simulink model "sl_lanechange"  (Simulink 7.5)
settings: Solver=ode45  StartTime=0.0  StopTime=10.0  RelTol=1e-3
libraries: simulink x2, roblocks x1
settings Model: Creator=pic  LastModifiedBy=corkep
settings DebuggingCC: StrictBusMsg=Warning

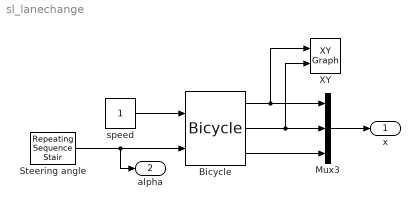
== system sl_lanechange ==
  Bicycle : roblocks/Bicycle  SystemSampleTime=-1  accel=1  vlim=1  alim=2  x0=[0, 0, 0]
  Mux3 : Mux  Inputs=3
  Steering angle : simulink/Sources/Repeating Sequence Stair  SystemSampleTime=-1  OutValues=[0 0 0 0.5 0 -0.5 0 0 0 0]  tsamp=1  OutMin=[]  OutMax=[]  OutDataTypeStr=double  OutputDataTypeScalingMode=Specify via dialog  OutDataType=double  ConRadixGroup=Best Precision: Vector-wise  OutScaling=2^-12
  XY : simulink/Sinks/XY Graph  SystemSampleTime=-1  xmin=0  xmax=10  ymin=0  ymax=10  st=-1
  speed : Constant  VectorParams1D=off  OutDataType=fixdt(1, 16)  OutScaling=2^0  SampleTime=0.02
  x : Outport  OutDataType=fixdt(1, 16)  OutScaling=2^0
  alpha : Outport  Port=2  OutDataType=fixdt(1, 16)  OutScaling=2^0
  wires:
  Steering angle/1 -> alpha/1, Bicycle/2
  speed/1 -> Bicycle/1
  Bicycle/3 -> Mux3/3
  Bicycle/1 -> Mux3/1, XY/1
  Bicycle/2 -> Mux3/2, XY/2
  Mux3/1 -> x/1
